simulink model "pmsm_model_lab2_Discrete_2025_st_R2020a"  (R2023a)
settings: Solver=ode23tb  StartTime=0.0  StopTime=1  FixedStep=0.0001  MaxStep=Tsim  RelTol=1e-3
values from neighbouring files (symbols this model uses):
  C32 = [ 1       0 ... (first row only)    [pmsm_param_Lab1_2025.m]    (also in pmsm_param_Lab2_2025_st.m; pmsm_param_Lab3_st.m; pmsm_param_Lab4_2024_st.m)
  C32inv = 2/3*[1    -1/2        -1/2 ... (first row only)    [pmsm_param_Lab1_2025.m]    (also in pmsm_param_Lab2_2025_st.m; pmsm_param_Lab3_st.m; pmsm_param_Lab4_2024_st.m)
  C33 = C32*C32inv    [pmsm_param_Lab1_2025.m]    (also in pmsm_param_Lab2_2025_st.m; pmsm_param_Lab3_st.m; pmsm_param_Lab4_2024_st.m)
  f = 15e-3    (= 0.015)    [pmsm_param_Lab1_2025.m]    (also in pmsm_param_Lab2_2025_st.m; pmsm_param_Lab3_st.m; pmsm_param_Lab4_2024_st.m)
  GVSI = 1    [pmsm_param_Lab2_2025_st.m]    (also in pmsm_param_Lab3_st.m; pmsm_param_Lab4_2024_st.m)
  Id0 = 0    [pmsm_param_Lab1_2025.m]    (also in pmsm_param_Lab2_2025_st.m; pmsm_param_Lab3_st.m = interp1(Tref,Idopt,Tm0); pmsm_param_Lab4_2024_st.m = interp1(Tref,Idopt,Tm0))
  Iq0 = 2/3*Tm0/(Pp*Psif)    (= 0)    [pmsm_param_Lab1_2025.m]    (also in pmsm_param_Lab2_2025_st.m = 119.926066866; pmsm_param_Lab3_st.m = interp1(Tref,Iqopt,Tm0); pmsm_param_Lab4_2024_st.m = interp1(Tref,Iqopt,Tm0))
  J = 100e-3    (= 0.1)    [pmsm_param_Lab1_2025.m]    (also in pmsm_param_Lab2_2025_st.m; pmsm_param_Lab3_st.m; pmsm_param_Lab4_2024_st.m)
  Kid = Kpd / tid    (= 180)    [pmsm_param_Lab2_2025_st.m]    (also in pmsm_param_Lab3_st.m; pmsm_param_Lab4_2024_st.m)
  Kiq = Kpq / tiq    (= 180)    [pmsm_param_Lab2_2025_st.m]    (also in pmsm_param_Lab3_st.m; pmsm_param_Lab4_2024_st.m)
  kL = 0.750    (= 0.75)    [pmsm_param_Lab1_2025.m]    (also in pmsm_param_Lab2_2025_st.m; pmsm_param_Lab3_st.m; pmsm_param_Lab4_2024_st.m)
  Kpd = (3*Ld0) / tr    (= 3)    [pmsm_param_Lab2_2025_st.m]    (also in pmsm_param_Lab3_st.m; pmsm_param_Lab4_2024_st.m)
  Kpq = (3 * Lq0) / tr    (= 6)    [pmsm_param_Lab2_2025_st.m]    (also in pmsm_param_Lab3_st.m; pmsm_param_Lab4_2024_st.m)
  Ld0 = 1.0*Ld    (= 0.001)    [pmsm_param_Lab2_2025_st.m]    (also in pmsm_param_Lab3_st.m; pmsm_param_Lab4_2024_st.m)
  Lq0 = 1.0*Lq    (= 0.002)    [pmsm_param_Lab2_2025_st.m]    (also in pmsm_param_Lab3_st.m; pmsm_param_Lab4_2024_st.m)
  Pp = 4    [pmsm_param_Lab1_2025.m]    (also in pmsm_param_Lab2_2025_st.m; pmsm_param_Lab3_st.m; pmsm_param_Lab4_2024_st.m)
  Psid0 = interpn(Idv,Iqv,Psidd,Id0,Iq0)    [pmsm_param_Lab1_2025.m]    (also in pmsm_param_Lab2_2025_st.m; pmsm_param_Lab3_st.m; pmsm_param_Lab4_2024_st.m)
  Psif0 = 1.0*Psif    (= 0.167)    [pmsm_param_Lab2_2025_st.m]    (also in pmsm_param_Lab3_st.m; pmsm_param_Lab4_2024_st.m)
  Psiq0 = interpn(Idv,Iqv,Psiqq,Id0,Iq0)    [pmsm_param_Lab1_2025.m]    (also in pmsm_param_Lab2_2025_st.m; pmsm_param_Lab3_st.m; pmsm_param_Lab4_2024_st.m)
  Rs = 60e-3    (= 0.06)    [pmsm_param_Lab1_2025.m]    (also in pmsm_param_Lab2_2025_st.m; pmsm_param_Lab3_st.m; pmsm_param_Lab4_2024_st.m)
  Thetae0 = 0    [pmsm_param_Lab1_2025.m]    (also in pmsm_param_Lab2_2025_st.m; pmsm_param_Lab3_st.m; pmsm_param_Lab4_2024_st.m)
  Ts = Tp    (= 0.0001)    [pmsm_param_Lab2_2025_st.m]    (also in pmsm_param_Lab3_st.m; pmsm_param_Lab4_2024_st.m)
  Ts_Dis = 1/fs    (= 0.0001)    [pmsm_param_Lab2_2025_st.m]
  Tstep = 0.10    (= 0.1)    [pmsm_param_Lab2_2025_st.m]    (also in pmsm_param_Lab3_st.m = 0.05; pmsm_param_Lab4_2024_st.m = 0.05)
  Ud0 = Rs*Id0    (= 0)    [pmsm_param_Lab2_2025_st.m]    (also in pmsm_param_Lab3_st.m; pmsm_param_Lab4_2024_st.m)
  Uq0 = Rs*Iq0    (= 7.19556401196)    [pmsm_param_Lab2_2025_st.m]    (also in pmsm_param_Lab3_st.m = 11.5129024191; pmsm_param_Lab4_2024_st.m = Rs*Iq0)
  Vd0 = Rs*Id0-Pp*Psiq0*Wm0    [pmsm_param_Lab1_2025.m]    (also in pmsm_param_Lab2_2025_st.m = Ud0-Pp*Psiq0*Wm0; pmsm_param_Lab3_st.m = Ud0-Pp*Psiq0*Wm0; pmsm_param_Lab4_2024_st.m = Ud0-Pp*Psiq0*Wm0)
  Vq0 = Rs*Iq0+Pp*Psid0*Wm0    [pmsm_param_Lab1_2025.m]    (also in pmsm_param_Lab2_2025_st.m = Uq0+Pp*Psid0*Wm0; pmsm_param_Lab3_st.m = Uq0+Pp*Psid0*Wm0; pmsm_param_Lab4_2024_st.m = Uq0+Pp*Psid0*Wm0)
  Wm0 = 0    [pmsm_param_Lab1_2025.m]    (also in pmsm_param_Lab2_2025_st.m = 157.079632679; pmsm_param_Lab3_st.m = 251.327412287; pmsm_param_Lab4_2024_st.m)
undefined symbols (not defined in the file or in its folder): Idd, Iqq, Psidv, Psiqv
settings Model: Creator=babak_  LastModifiedBy=Henry
settings SolverCC: AlgebraicLoopSolver=LineSearch
settings DataIOCC: LimitDataPoints=on  SaveFormat=Array  SignalLoggingSaveFormat=ModelDataLogs  ReturnWorkspaceOutputs=off
settings OptimizationCC: BooleanDataType=off  ExpressionDepthLimit=2147483647  InitFltsAndDblsToZero=on  LifeSpan=inf
settings DebuggingCC: SaveWithParameterizedLinksMsg=none  UnderspecifiedInitializationDetection=Classic  MergeDetectMultiDrivingBlocksExec=none  SignalResolutionControl=TryResolveAllWithWarning  MultiTaskDSMMsg=warning  MultiTaskCondExecSysMsg=none  FcnCallInpInsideContextMsg=warning  UnconnectedInputMsg=warning  UnconnectedOutputMsg=warning  UnconnectedLineMsg=warning  StateNameClashWarn=warning  SFUnexpectedBacktrackingDiag=warning  SFNoUnconditionalDefaultTransitionDiag=warning  ArithmeticOperatorsInVariantConditions=warning
settings HardwareCC: ProdBitPerPointer=32  ProdBitPerSizeT=32  ProdBitPerPtrDiffT=32  ProdLargestAtomicFloat=None  ProdIntDivRoundTo=Undefined  ProdEndianess=Unspecified  ProdWordSize=32  ProdHWDeviceType=32-bit Generic  TargetUnknown=on
settings ModelReferenceCC: EnableRefExpFcnMdlSchedulingChecks=on  PropagateSignalLabelsOutOfModel=off
settings SFSimCC: SimUseLocalCustomCode=off  CustomCodeUndefinedFunction=UseInterfaceOnly
settings RTWCC: RTWUseLocalCustomCode=off
settings CodeAppCC: StateflowObjectComments=on
settings GRTTargetCC: TargetFcnLib=ansi_tfl_tmw.mat  TargetLangStandard=C89/C90 (ANSI)  ModelReferenceCompliant=off  CompOptLevelCompliant=off  CombineOutputUpdateFcns=off  MatFileLogging=off  GRTInterface=on
settings ConfigComp: CovMetricSettings=dw  CovSaveCumulativeToWorkspaceVar=on  CovSaveSingleToWorkspaceVar=on  CovExternalEMLEnable=off

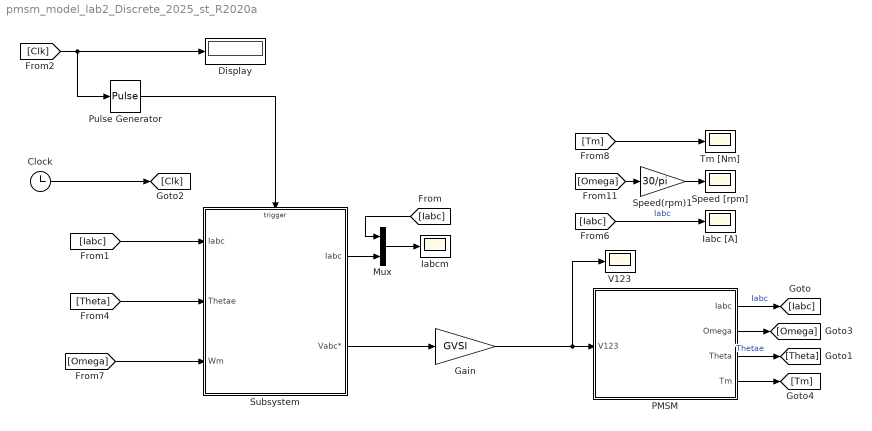
== system pmsm_model_lab2_Discrete_2025_st_R2020a ==
  Clock : Clock
  Display : Display
  Gain : Gain  Gain=GVSI
  Iabc [A] : Scope
  Iabcm : Scope
  Mux : Mux  Inputs=2
  PMSM : Subsystem
  Pulse Generator : DiscretePulseGenerator  PulseType=Time based  TimeSource=Use external signal  Period=Ts_Dis  PulseWidth=5
  Speed [rpm] : Scope
  Speed(rpm)1 : Gain  Gain=30/pi
  Subsystem : Subsystem
  Tm [Nm] : Scope
  "V123 " : Scope
  wires:
  PMSM/3(Theta) -> [Theta]  "Thetae"
  PMSM/4(Tm) -> [Tm]
  Clock/1 -> [Clk]
  PMSM/1(Iabc) -> [Iabc]  "Iabc"
  Mux/1 -> Iabcm/1
  [Iabc] -> Mux/1
  Gain/1 -> PMSM/1(V123), "V123 "/1
  Speed(rpm)1/1 -> Speed [rpm]/1
  [Omega] -> Speed(rpm)1/1
  [Tm] -> Tm [Nm]/1
  [Iabc] -> Iabc [A]/1  "Iabc"
  PMSM/2(Omega) -> [Omega]
  [Clk] -> Pulse Generator/1, Display/1
  [Iabc] -> Subsystem/1(Iabc)
  [Theta] -> Subsystem/2(Thetae)
  [Omega] -> Subsystem/3(Wm)
  Subsystem/1("Iabc ") -> Mux/2
  Subsystem/2(Vabc*) -> Gain/1
  Pulse Generator/1 -> Subsystem/Trigger

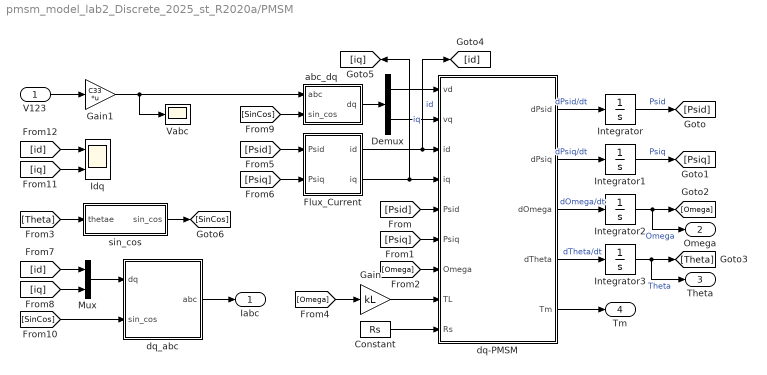
== system pmsm_model_lab2_Discrete_2025_st_R2020a/PMSM ==
  V123 : Inport
  Constant : Constant  Value=Rs
  Demux : Demux  Outputs=2
  Flux_Current : Subsystem
  Gain : Gain  Gain=kL
  Gain1 : Gain  Gain=C33  Multiplication=Matrix(K*u)
  Idq : Scope  NumInputPorts=2
  Integrator : Integrator  InitialCondition=Psid0
  Integrator1 : Integrator  InitialCondition=Psiq0
  Integrator2 : Integrator  InitialCondition=Wm0
  Integrator3 : Integrator  InitialCondition=Thetae0
  Mux : Mux  Inputs=2
  Vabc : Scope
  abc_dq : Subsystem
  dq-PMSM : MATLAB Function  TreatAsAtomicUnit=on
  dq_abc : Subsystem
  sin_cos : Subsystem
  Iabc : Outport
  Omega : Outport  Port=2
  Theta : Outport  Port=3
  Tm : Outport  Port=4
  wires:
  dq-PMSM/1(dPsid) -> Integrator/1  "dPsid/dt"
  dq-PMSM/2(dPsiq) -> Integrator1/1  "dPsiq/dt"
  Integrator3/1 -> [Theta], Theta/1  "Theta"
  [Omega] -> Gain/1
  Flux_Current/1(id) -> [id], dq-PMSM/3(id)  "id"
  [SinCos] -> dq_abc/2(sin_cos)
  Integrator1/1 -> [Psiq]  "Psiq"
  sin_cos/1(sin_cos) -> [SinCos]
  dq_abc/1(abc) -> Iabc/1
  dq-PMSM/4(dTheta) -> Integrator3/1  "dTheta/dt"
  Demux/1 -> dq-PMSM/1(vd)
  [iq] -> Mux/2
  Mux/1 -> dq_abc/1(dq)
  dq-PMSM/3(dOmega) -> Integrator2/1  "dOmega/dt"
  [Psiq] -> dq-PMSM/6(Psiq)
  [Psid] -> dq-PMSM/5(Psid)
  [Theta] -> sin_cos/1(thetae)
  abc_dq/1(dq) -> Demux/1
  [SinCos] -> abc_dq/2(sin_cos)
  Gain/1 -> dq-PMSM/8(TL)
  Demux/2 -> dq-PMSM/2(vq)
  [Omega] -> dq-PMSM/7(Omega)
  V123/1 -> Gain1/1
  [id] -> Mux/1
  Integrator2/1 -> [Omega], Omega/1  "Omega"
  Flux_Current/2(iq) -> dq-PMSM/4(iq), [iq]  "iq"
  Integrator/1 -> [Psid]  "Psid"
  Constant/1 -> dq-PMSM/9(Rs)
  Gain1/1 -> abc_dq/1(abc), Vabc/1
  dq-PMSM/5(Tm) -> Tm/1
  [id] -> Idq/1
  [iq] -> Idq/2
  [Psid] -> Flux_Current/1(Psid)
  [Psiq] -> Flux_Current/2(Psiq)

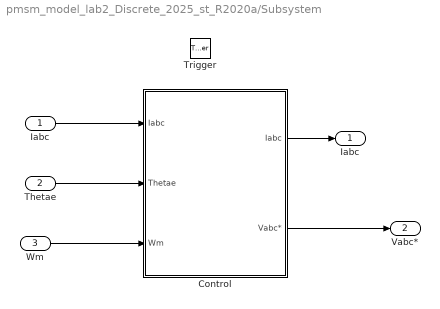
== system pmsm_model_lab2_Discrete_2025_st_R2020a/Subsystem ==
  Iabc : Inport
  Thetae : Inport  Port=2
  Wm : Inport  Port=3
  Trigger : TriggerPort  VariantControl=(inherit)  PortDimensions=1
  Control : Subsystem
  "Iabc " : Outport
  Vabc* : Outport  Port=2
  wires:
  Wm/1 -> Control/3(Wm)
  Control/2(Vabc*) -> Vabc*/1
  Control/1("Iabc ") -> "Iabc "/1
  Iabc/1 -> Control/1(Iabc)
  Thetae/1 -> Control/2(Thetae)

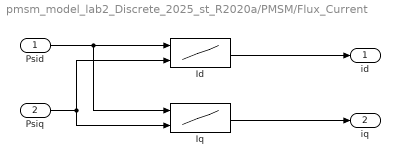
== system pmsm_model_lab2_Discrete_2025_st_R2020a/PMSM/Flux_Current ==
  Psid : Inport
  Psiq : Inport  Port=2
  Id : Lookup_n-D  BreakpointsForDimension1=Psidv  BreakpointsForDimension2=Psiqv  Table=Idd  InternalRulePriority=Speed  RndMeth=Simplest
      settings: InputPortMap=u0,u1
  Iq : Lookup_n-D  BreakpointsForDimension1=Psidv  BreakpointsForDimension2=Psiqv  Table=Iqq  InternalRulePriority=Speed  RndMeth=Simplest
      settings: InputPortMap=u0,u1
  id : Outport
  iq : Outport  Port=2
  wires:
  Psiq/1 -> Iq/2, Id/2
  Psid/1 -> Iq/1, Id/1
  Iq/1 -> iq/1
  Id/1 -> id/1

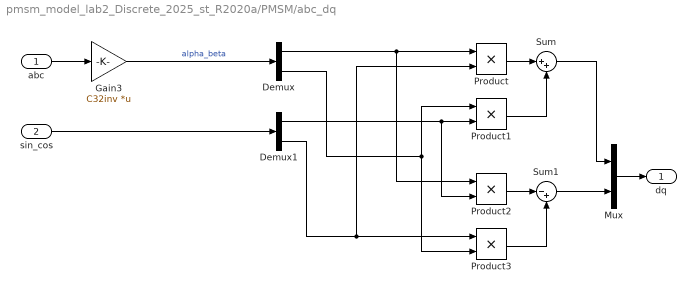
== system pmsm_model_lab2_Discrete_2025_st_R2020a/PMSM/abc_dq ==
  abc : Inport
  sin_cos : Inport  Port=2
  Demux : Demux  Outputs=2
      settings: DisplayOption=none
  Demux1 : Demux  Outputs=2
      settings: DisplayOption=none
  Gain3 : Gain  Gain=C32inv  Multiplication=Matrix(K*u)  OutDataTypeStr=Inherit: Same as input  ParamDataTypeStr=Inherit: Same as input
  Mux : Mux  Inputs=2
  Product{,1..3} (4 alike) : Product  InputSameDT=on  RndMeth=Zero  SaturateOnIntegerOverflow=on  OutDataTypeStr=Inherit: Same as first input
  Sum : Sum  Inputs=|++  InputSameDT=on  SaturateOnIntegerOverflow=on  OutDataTypeStr=Inherit: Same as first input
  Sum1 : Sum  Inputs=|-+  InputSameDT=on  SaturateOnIntegerOverflow=on  OutDataTypeStr=Inherit: Same as first input
  dq : Outport
  wires:
  Sum1/1 -> Mux/2
  Mux/1 -> dq/1
  Demux1/1 -> Product2/2, Product1/2
  sin_cos/1 -> Demux1/1
  Demux/2 -> Product3/2, Product1/1
  Gain3/1 -> Demux/1  "alpha_beta"
  abc/1 -> Gain3/1
  Demux1/2 -> Product3/1, Product/2
  Demux/1 -> Product2/1, Product/1
  Sum/1 -> Mux/1
  Product3/1 -> Sum1/2
  Product2/1 -> Sum1/1
  Product1/1 -> Sum/2
  Product/1 -> Sum/1

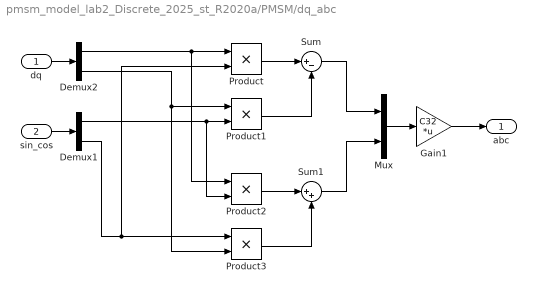
== system pmsm_model_lab2_Discrete_2025_st_R2020a/PMSM/dq_abc ==
  dq : Inport
  sin_cos : Inport  Port=2
  Demux1 : Demux  Outputs=2
      settings: DisplayOption=none
  Demux2 : Demux  Outputs=2
      settings: DisplayOption=none
  Gain1 : Gain  Gain=C32  Multiplication=Matrix(K*u)  OutDataTypeStr=Inherit: Same as input  ParamDataTypeStr=Inherit: Same as input
  Mux : Mux  Inputs=2
  Product{,1..3} (4 alike) : Product  InputSameDT=on  RndMeth=Zero  SaturateOnIntegerOverflow=on  OutDataTypeStr=Inherit: Same as first input
  Sum : Sum  Inputs=|+-  InputSameDT=on  SaturateOnIntegerOverflow=on  OutDataTypeStr=Inherit: Same as first input
  Sum1 : Sum  Inputs=|++  InputSameDT=on  SaturateOnIntegerOverflow=on  OutDataTypeStr=Inherit: Same as first input
  abc : Outport
  wires:
  Mux/1 -> Gain1/1
  Demux1/1 -> Product2/2, Product1/2
  sin_cos/1 -> Demux1/1
  dq/1 -> Demux2/1
  Demux1/2 -> Product3/1, Product/2
  Product3/1 -> Sum1/2
  Product2/1 -> Sum1/1
  Product1/1 -> Sum/2
  Product/1 -> Sum/1
  Demux2/1 -> Product/1, Product2/1
  Demux2/2 -> Product3/2, Product1/1
  Sum/1 -> Mux/1
  Sum1/1 -> Mux/2
  Gain1/1 -> abc/1

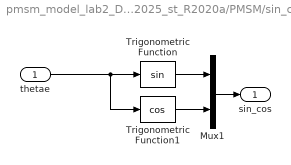
== system pmsm_model_lab2_Discrete_2025_st_R2020a/PMSM/sin_cos ==
  thetae : Inport
  Mux1 : Mux  Inputs=2
  Trigonometric Function : Trigonometry
  Trigonometric Function1 : Trigonometry  Operator=cos
  sin_cos : Outport
  wires:
  Trigonometric Function/1 -> Mux1/1
  Trigonometric Function1/1 -> Mux1/2
  thetae/1 -> Trigonometric Function1/1, Trigonometric Function/1
  Mux1/1 -> sin_cos/1

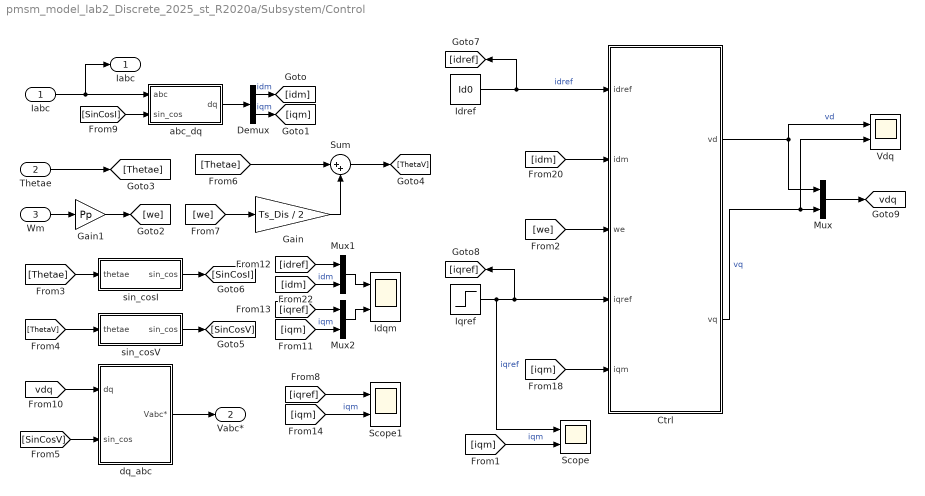
== system pmsm_model_lab2_Discrete_2025_st_R2020a/Subsystem/Control ==
  Iabc : Inport
  Thetae : Inport  Port=2
  Wm : Inport  Port=3
  Ctrl : MATLAB Function  TreatAsAtomicUnit=on
  Demux : Demux  Outputs=2
  Gain : Gain  Gain=Ts_Dis / 2
  Gain1 : Gain  Gain=Pp
  Idqm : Scope  NumInputPorts=2
  Idref : Constant  Value=Id0
  Iqref : Step  Time=Tstep  Before=Iq0  After=Iq0+10
  Mux : Mux  Inputs=2
  Mux1 : Mux  Inputs=2
  Mux2 : Mux  Inputs=2
  Scope : Scope  NumInputPorts=2
  Scope1 : Scope  NumInputPorts=2
  Sum : Sum  Inputs=|++
  Vdq : Scope  NumInputPorts=2
  abc_dq : Subsystem
  dq_abc : Subsystem
  sin_cosI : Subsystem
  sin_cosV : Subsystem
  "Iabc " : Outport
  Vabc* : Outport  Port=2
  tag scope: vdq=global
  wires:
  [SinCosI] -> abc_dq/2(sin_cos)
  sin_cosI/1(sin_cos) -> [SinCosI]
  [SinCosV] -> dq_abc/2(sin_cos)
  Ctrl/2(vq) -> Mux/2, Vdq/2  "vq"
  Ctrl/1(vd) -> Mux/1, Vdq/1  "vd"
  [Thetae] -> sin_cosI/1(thetae)
  [ThetaV] -> sin_cosV/1(thetae)
  sin_cosV/1(sin_cos) -> [SinCosV]
  Sum/1 -> [ThetaV]
  [Thetae] -> Sum/1
  [we] -> Gain/1
  Gain/1 -> Sum/2
  Iabc/1 -> "Iabc "/1, abc_dq/1(abc)
  Gain1/1 -> [we]
  [iqm] -> Mux2/2  "iqm"
  Iqref/1 -> Scope/1, [iqref], Ctrl/4(iqref)  "iqref"
  Demux/1 -> [idm]  "idm"
  [idm] -> Mux1/2  "idm"
  Demux/2 -> [iqm]  "iqm"
  Idref/1 -> Ctrl/1(idref), [idref]  "idref"
  Mux2/1 -> Idqm/2
  Mux1/1 -> Idqm/1
  abc_dq/1(dq) -> Demux/1
  Mux/1 -> [vdq]
  [vdq] -> dq_abc/1(dq)
  Wm/1 -> Gain1/1
  Thetae/1 -> [Thetae]
  [idref] -> Mux1/1
  [iqref] -> Mux2/1
  dq_abc/1(Vabc*) -> Vabc*/1
  [idm] -> Ctrl/2(idm)
  [we] -> Ctrl/3(we)
  [iqm] -> Ctrl/5(iqm)
  [iqm] -> Scope/2  "iqm"
  [iqref] -> Scope1/1
  [iqm] -> Scope1/2  "iqm"

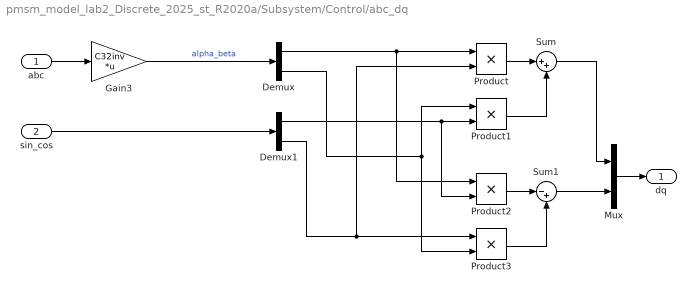
== system pmsm_model_lab2_Discrete_2025_st_R2020a/Subsystem/Control/abc_dq ==
  abc : Inport
  sin_cos : Inport  Port=2
  Demux : Demux  Outputs=2
      settings: DisplayOption=none
  Demux1 : Demux  Outputs=2
      settings: DisplayOption=none
  Gain3 : Gain  Gain=C32inv  Multiplication=Matrix(K*u)  OutDataTypeStr=Inherit: Same as input  ParamDataTypeStr=Inherit: Same as input
  Mux : Mux  Inputs=2
  Product{,1..3} (4 alike) : Product  InputSameDT=on  RndMeth=Zero  SaturateOnIntegerOverflow=on  OutDataTypeStr=Inherit: Same as first input
  Sum : Sum  Inputs=|++  InputSameDT=on  SaturateOnIntegerOverflow=on  OutDataTypeStr=Inherit: Same as first input
  Sum1 : Sum  Inputs=|-+  InputSameDT=on  SaturateOnIntegerOverflow=on  OutDataTypeStr=Inherit: Same as first input
  dq : Outport
  wires:
  Product/1 -> Sum/1
  Product1/1 -> Sum/2
  Product2/1 -> Sum1/1
  Product3/1 -> Sum1/2
  Sum/1 -> Mux/1
  Demux/1 -> Product/1, Product2/1
  Demux1/2 -> Product/2, Product3/1
  abc/1 -> Gain3/1
  Gain3/1 -> Demux/1  "alpha_beta"
  Demux/2 -> Product1/1, Product3/2
  sin_cos/1 -> Demux1/1
  Demux1/1 -> Product1/2, Product2/2
  Mux/1 -> dq/1
  Sum1/1 -> Mux/2

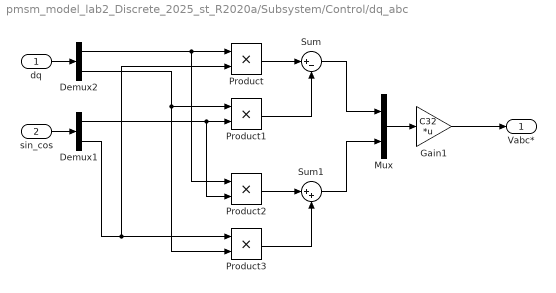
== system pmsm_model_lab2_Discrete_2025_st_R2020a/Subsystem/Control/dq_abc ==
  dq : Inport
  sin_cos : Inport  Port=2
  Demux1 : Demux  Outputs=2
      settings: DisplayOption=none
  Demux2 : Demux  Outputs=2
      settings: DisplayOption=none
  Gain1 : Gain  Gain=C32  Multiplication=Matrix(K*u)  OutDataTypeStr=Inherit: Same as input  ParamDataTypeStr=Inherit: Same as input
  Mux : Mux  Inputs=2
  Product{,1..3} (4 alike) : Product  InputSameDT=on  RndMeth=Zero  SaturateOnIntegerOverflow=on  OutDataTypeStr=Inherit: Same as first input
  Sum : Sum  Inputs=|+-  InputSameDT=on  SaturateOnIntegerOverflow=on  OutDataTypeStr=Inherit: Same as first input
  Sum1 : Sum  Inputs=|++  InputSameDT=on  SaturateOnIntegerOverflow=on  OutDataTypeStr=Inherit: Same as first input
  Vabc* : Outport
  wires:
  Sum1/1 -> Mux/2
  Sum/1 -> Mux/1
  Demux2/2 -> Product1/1, Product3/2
  Demux2/1 -> Product2/1, Product/1
  Product/1 -> Sum/1
  Product1/1 -> Sum/2
  Product2/1 -> Sum1/1
  Product3/1 -> Sum1/2
  Demux1/2 -> Product/2, Product3/1
  sin_cos/1 -> Demux1/1
  Demux1/1 -> Product1/2, Product2/2
  Mux/1 -> Gain1/1
  dq/1 -> Demux2/1
  Gain1/1 -> Vabc*/1

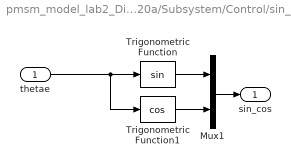
== system pmsm_model_lab2_Discrete_2025_st_R2020a/Subsystem/Control/sin_cosI ==
  thetae : Inport
  Mux1 : Mux  Inputs=2
  Trigonometric Function : Trigonometry
  Trigonometric Function1 : Trigonometry  Operator=cos
  sin_cos : Outport
  wires:
  Mux1/1 -> sin_cos/1
  thetae/1 -> Trigonometric Function/1, Trigonometric Function1/1
  Trigonometric Function1/1 -> Mux1/2
  Trigonometric Function/1 -> Mux1/1

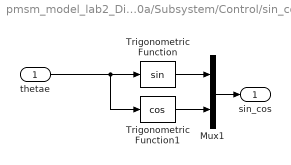
== system pmsm_model_lab2_Discrete_2025_st_R2020a/Subsystem/Control/sin_cosV ==
  thetae : Inport
  Mux1 : Mux  Inputs=2
  Trigonometric Function : Trigonometry
  Trigonometric Function1 : Trigonometry  Operator=cos
  sin_cos : Outport
  wires:
  Mux1/1 -> sin_cos/1
  thetae/1 -> Trigonometric Function/1, Trigonometric Function1/1
  Trigonometric Function1/1 -> Mux1/2
  Trigonometric Function/1 -> Mux1/1

== matlab function pmsm_model_lab2_Discrete_2025_st_R2020a/PMSM/dq-PMSM ==
  data: vd input; dPsid output; vq input; id input; iq input; Psid input; Psiq input; Omega input; TL input; dPsiq output; dOmega output; dTheta output; Rs input; Pp parameter; f parameter; J parameter; Tm output
function [dPsid, dPsiq, dOmega, dTheta, Tm] = PMSM(vd, vq, id, iq, Psid, Psiq, Omega, TL, Rs, Pp, f, J)

w=Pp*Omega;
Tm=(3/2)*Pp*(Psid*iq-Psiq*id);   % Clarke
% Tm=p*(Psid*iq-Psiq*id);       % Concordia

dPsid=vd-Rs*id+w*Psiq;
dPsiq=vq-Rs*iq-w*Psid;
dOmega=(Tm-f*Omega-TL)/J;
dTheta=w;

== matlab function pmsm_model_lab2_Discrete_2025_st_R2020a/Subsystem/Control/Ctrl ==
  settings: updateMethod=DISCRETE
  data: idref input; idm input; we input; iqref input; iqm input; Psif0 parameter; Ld0 parameter; Lq0 parameter; vd output; vq output; Kpd parameter; Kpq parameter; Kid parameter; Kiq parameter; Vd0 parameter; Vq0 parameter; Ud0 parameter; Uq0 parameter; Ts parameter
function [vd, vq]  = Ctrl(idref, idm, we, iqref, iqm, Psif0, Ld0, Lq0, Kpd, Kpq, Kid, Kiq, Vd0, Vq0, Ud0, Uq0, Ts)

persistent interrd interrq 

if isempty(interrd), interrd = Ud0; end
if isempty(interrq), interrq = Uq0; end

%error Calculation
errd= idref - idm;
errq= iqref - iqm;


%Integration Part
interrd= interrd + (Kid * errd * Ts);
interrq= interrq + (Kiq * errq * Ts);


%Control Voltage Calculation
vd= ((Kpd * errd) + interrd) - (Lq0 * we * iqm);
vq= ((Kpq * errq) + interrq)+  (Ld0 * we * idm) + (Psif0 * we);
